simulink model "abs_11"  (R2021a)
settings: Solver=VariableStepAuto  StartTime=0.0  StopTime=10.0  RelTol=1e-3
settings Model: Creator=yasso  LastModifiedBy=yasso

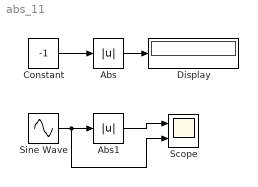
== system abs_11 ==
  Abs : Abs
  Abs1 : Abs
  Constant : Constant  Value=-1
  Display : Display
  Scope : Scope  NumInputPorts=2
  Sine Wave : Sin  SampleTime=0
  wires:
  Constant/1 -> Abs/1
  Abs/1 -> Display/1
  Sine Wave/1 -> Scope/2, Abs1/1
  Abs1/1 -> Scope/1
